simulink model "Lab3SquareDrive"  (R2024a)
settings: Solver=FixedStepDiscrete  StartTime=0.0  StopTime=90  FixedStep=0.01  RelTol=1e-3
undefined symbols (not defined in the file): DiscIntNeverNeededParam
libraries: mobileRoboticsTrainingLib x1
settings Model: PacingRate=5  Creator=Beast  LastModifiedBy=Beast

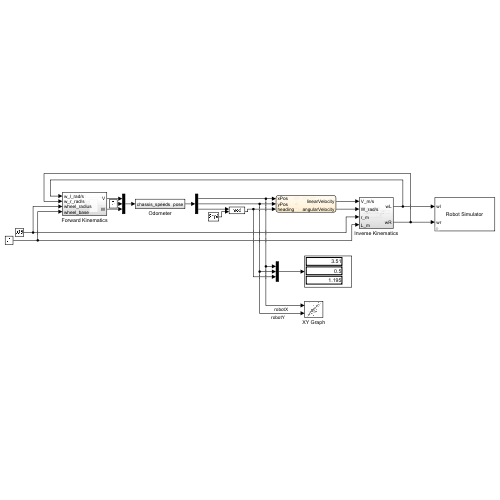
[thumbnail: Simulink's stored preview of the top-level diagram]
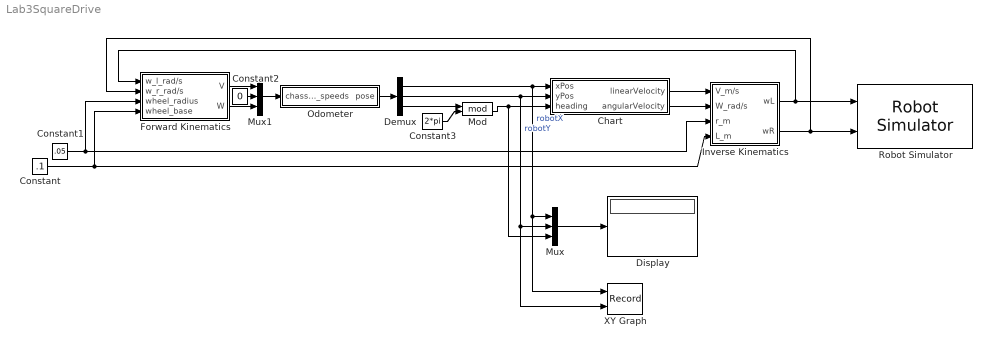
== system Lab3SquareDrive ==
  Chart : Stateflow chart  TreatAsAtomicUnit=on
  Constant : Constant  Value=.1
  Constant1 : Constant  Value=.05
  Constant2 : Constant  Value=0
  Constant3 : Constant  Value=2*pi
  Demux : Demux  Outputs=3
  Display : Display
  Forward Kinematics : Subsystem
  Inverse Kinematics : Subsystem
  Mod : Math  Operator=mod
  Mux : Mux  Inputs=3
  Mux1 : Mux  Inputs=3
  Odometer : Subsystem
  Robot Simulator : mobileRoboticsTrainingLib/Robot Simulator  Priority=99  mapVar=[]  startX=.5  startY=.5  startTheta=0  axleLength=0.1  wheelR=0.05
  XY Graph : Record  FileSettingsInternal="{\"entries\":[{\"content\":{\"excelSettings\":{\"content\":{},\"type\":\"Streamout.ExcelSettings\"}},\"type\":\"Streamout.FileSettingStorage\",\"uuid\":\"\"}],\"packageUris\":[\"http:\\/\\/schema.mathworks.com\\/mf0\\/streamout_blocks\\/R2020a\"],\"version\":\"1.0\"}"  Layout=[1 1]  SignalsInternal="{\"entries\":[{\"content\":{\"signals\":[{\"content\":{\"blockPath\":[],\"dimensions\":[1],\"domain\":\"\",\"lineColor\":\"#a2142f\",\"plots\":[ 1 ],\"port\":1,\"sid\":[\"\"],\"signalID\":1,\"signalName\":\"robotX\"},\"type\":\"RecordBlkView.Signal\",\"uuid\":\"\"},{\"content\":{\"blockPath\":[],\"dimensions\":[1],\"domain\":\"\",\"lineColor\":\"#139fff\",\"plots\":[ 1 ],\"port\":2,\"sid\":[\"\"],\"signalID\":2,\"signalName\":\"robotY\"},\"type\":\"RecordBlkView.Signal\",\"uuid\":\"\"}]},\"type\":\"RecordBlkView.InputSignals\",\"uuid\":\"\"}],\"packageUris\":[\"http:\\/\\/schema.mathworks.com\\/mf0\\/streamout_blocks\\/R2020a\"],\"version\":\"1.0\"}"  VisualizationBindings="{\"xyplotplugin\":{\"info\":[{\"series\":[{\"bindingParametersList\":[{\"parameter\":\"X-Axis\",\"signalID\":1,\"signalName\":\"robotX\"},{\"parameter\":\"Y-Axis\",\"signalID\":2,\"signalName\":\"robotY\"}],\"seriesID\":0}],\"subplotID\":1}]}}"  CompatibilityTag=XY
  wires:
  Chart/1(linearVelocity) -> Inverse Kinematics/1(V_m/s)
  Chart/2(angularVelocity) -> Inverse Kinematics/2(W_rad/s)
  Constant/1 -> Forward Kinematics/4(wheel_base), Inverse Kinematics/4(L_m)
  Constant1/1 -> Forward Kinematics/3(wheel_radius), Inverse Kinematics/3(r_m)
  Demux/1 -> XY Graph/1, Mux/1, Chart/1(xPos)  "robotX"
  Forward Kinematics/1(V) -> Mux1/1
  Forward Kinematics/2(W) -> Mux1/3
  Demux/2 -> XY Graph/2, Mux/2, Chart/2(yPos)  "robotY"
  Mux/1 -> Display/1
  Mux1/1 -> Odometer/1(chassis_speeds)
  Odometer/1(pose) -> Demux/1
  Constant2/1 -> Mux1/2
  Inverse Kinematics/1(wL) -> Forward Kinematics/1(w_l_rad/s), Robot Simulator/1
  Inverse Kinematics/2(wR) -> Forward Kinematics/2(w_r_rad/s), Robot Simulator/2
  Constant3/1 -> Mod/2
  Mod/1 -> Mux/3, Chart/3(heading)
  Demux/3 -> Mod/1

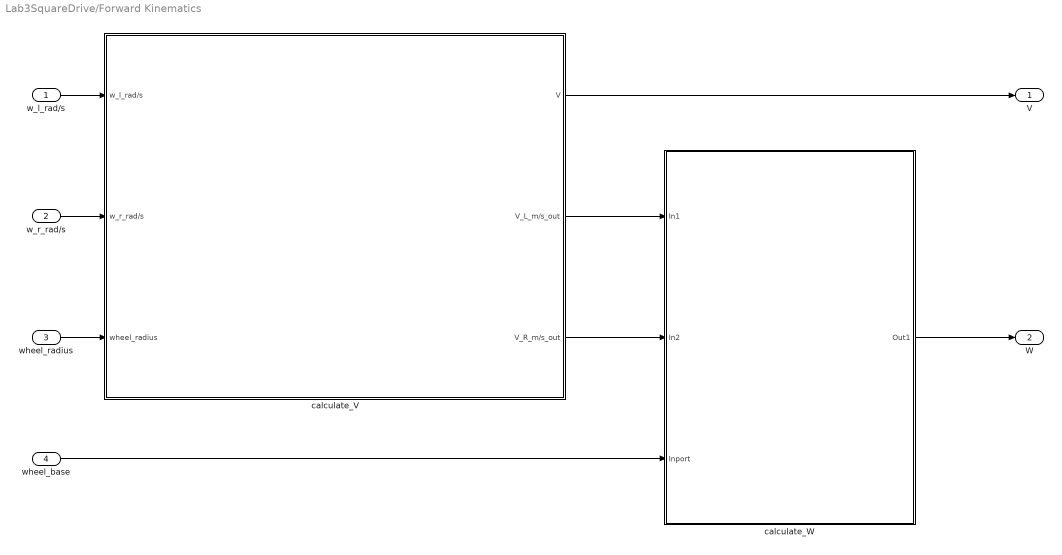
== system Lab3SquareDrive/Forward Kinematics ==
  w_l_rad/s : Inport
  w_r_rad/s : Inport  Port=2
  wheel_radius : Inport  Port=3
  wheel_base : Inport  Port=4
  calculate_V : Subsystem
  calculate_W : Subsystem
  V : Outport
  W : Outport  Port=2
  wires:
  calculate_V/1(V) -> V/1
  w_r_rad/s/1 -> calculate_V/2(w_r_rad/s)
  w_l_rad/s/1 -> calculate_V/1(w_l_rad/s)
  calculate_V/2(V_L_m/s_out) -> calculate_W/1(In1)
  calculate_W/1(Out1) -> W/1
  calculate_V/3(V_R_m/s_out) -> calculate_W/2(In2)
  wheel_radius/1 -> calculate_V/3(wheel_radius)
  wheel_base/1 -> calculate_W/3(Inport)

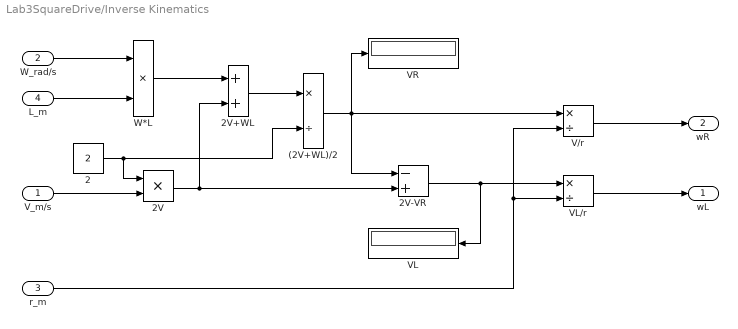
== system Lab3SquareDrive/Inverse Kinematics ==
  V_m/s : Inport
  W_rad/s : Inport  Port=2
  r_m : Inport  Port=3
  L_m : Inport  Port=4
  (2V+WL)/2 : Product  Inputs=*/
  2 : Constant  Value=2
  2V : Product
  2V+WL : Sum
  2V-VR : Sum  Inputs=-+
  V/r : Product  Inputs=*/
  VL : Display
  VL/r : Product  Inputs=*/
  VR : Display
  W*L : Product
  wL : Outport
  wR : Outport  Port=2
  wires:
  2/1 -> 2V/1, (2V+WL)/2/2
  W*L/1 -> 2V+WL/1
  (2V+WL)/2/1 -> 2V-VR/1, V/r/1, VR/1
  r_m/1 -> V/r/2, VL/r/2
  2V-VR/1 -> VL/r/1, VL/1
  2V/1 -> 2V+WL/2, 2V-VR/2
  VL/r/1 -> wL/1
  2V+WL/1 -> (2V+WL)/2/1
  V/r/1 -> wR/1
  V_m/s/1 -> 2V/2
  W_rad/s/1 -> W*L/1
  L_m/1 -> W*L/2

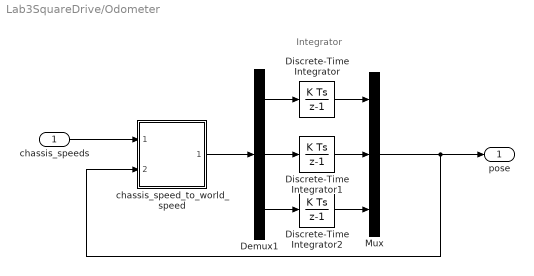
== system Lab3SquareDrive/Odometer ==
  note: Integrator
  chassis_speeds : Inport
  Demux1 : Demux  Outputs=3
  Discrete-Time Integrator : DiscreteIntegrator  InitialCondition=.5  SampleTime=-1  ICPrevOutput=DiscIntNeverNeededParam  ICPrevScaledInput=DiscIntNeverNeededParam
  Discrete-Time Integrator1 : DiscreteIntegrator  InitialCondition=.5  SampleTime=-1  ICPrevOutput=DiscIntNeverNeededParam  ICPrevScaledInput=DiscIntNeverNeededParam
  Discrete-Time Integrator2 : DiscreteIntegrator  SampleTime=-1  ICPrevOutput=DiscIntNeverNeededParam  ICPrevScaledInput=DiscIntNeverNeededParam
  Mux : Mux  Inputs=3
  chassis_speed_to_world_speed : Subsystem
  pose : Outport  VectorParamsAs1DForOutWhenUnconnected=off
  wires:
  Discrete-Time Integrator/1 -> Mux/1
  Demux1/2 -> Discrete-Time Integrator1/1
  Discrete-Time Integrator2/1 -> Mux/3
  Mux/1 -> chassis_speed_to_world_speed/2(last_pose), pose/1
  Demux1/3 -> Discrete-Time Integrator2/1
  Discrete-Time Integrator1/1 -> Mux/2
  Demux1/1 -> Discrete-Time Integrator/1
  chassis_speed_to_world_speed/1(global_velocity) -> Demux1/1
  chassis_speeds/1 -> chassis_speed_to_world_speed/1(robot_velocity)

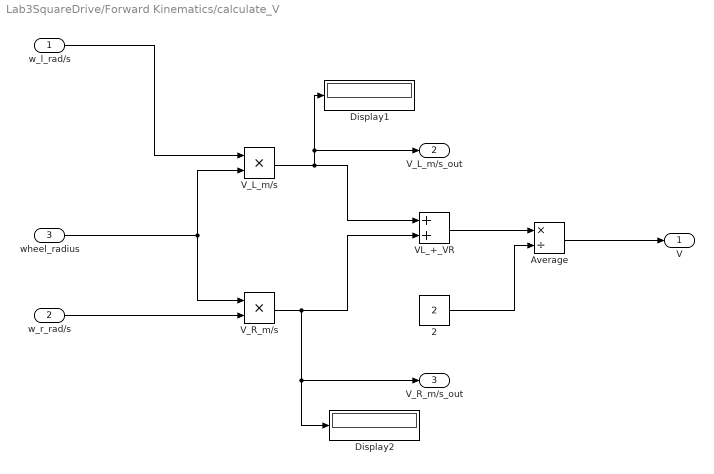
== system Lab3SquareDrive/Forward Kinematics/calculate_V ==
  w_l_rad/s : Inport
  w_r_rad/s : Inport  Port=2
  wheel_radius : Inport  Port=3
  2 : Constant  Value=2
  Average : Product  Inputs=*/
  Display1 : Display
  Display2 : Display
  VL_+_VR : Sum
  V_L_m/s : Product
  V_R_m/s : Product
  V : Outport
  V_L_m/s_out : Outport  Port=2
  V_R_m/s_out : Outport  Port=3
  wires:
  w_r_rad/s/1 -> V_R_m/s/2
  VL_+_VR/1 -> Average/1
  wheel_radius/1 -> V_L_m/s/2, V_R_m/s/1
  V_L_m/s/1 -> Display1/1, V_L_m/s_out/1, VL_+_VR/1
  V_R_m/s/1 -> V_R_m/s_out/1, Display2/1, VL_+_VR/2
  2/1 -> Average/2
  w_l_rad/s/1 -> V_L_m/s/1
  Average/1 -> V/1

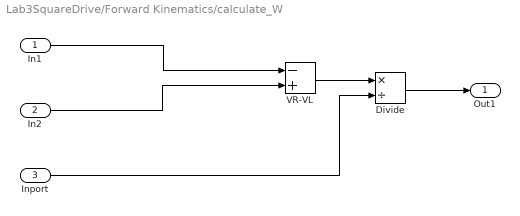
== system Lab3SquareDrive/Forward Kinematics/calculate_W ==
  In1 : Inport
  In2 : Inport  Port=2
  Inport : Inport  Port=3
  Divide : Product  Inputs=*/
  VR-VL : Sum  Inputs=-+
  Out1 : Outport
  wires:
  Inport/1 -> Divide/2
  VR-VL/1 -> Divide/1
  In2/1 -> VR-VL/2
  In1/1 -> VR-VL/1
  Divide/1 -> Out1/1

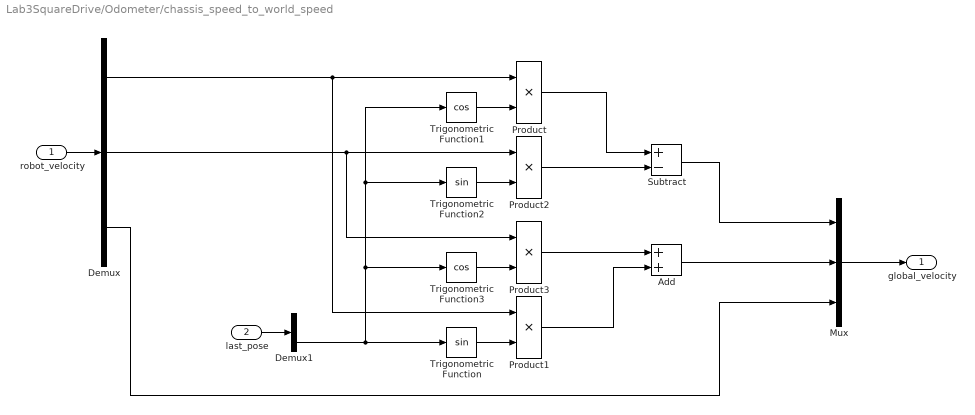
== system Lab3SquareDrive/Odometer/chassis_speed_to_world_speed ==
  robot_velocity : Inport
  last_pose : Inport  Port=2
  Add : Sum
  Demux : Demux  Outputs=3
  Demux1 : Demux  Outputs=3
  Mux : Mux  Inputs=3
  Product{,1..3} (4 alike) : Product
  Subtract : Sum  Inputs=+-
  Trigonometric Function : Trigonometry
  Trigonometric Function1 : Trigonometry  Operator=cos
  Trigonometric Function2 : Trigonometry
  Trigonometric Function3 : Trigonometry  Operator=cos
  global_velocity : Outport  VectorParamsAs1DForOutWhenUnconnected=off
  wires:
  Demux1/3 -> Trigonometric Function1/1, Trigonometric Function2/1, Trigonometric Function3/1, Trigonometric Function/1
  Trigonometric Function3/1 -> Product3/2
  Trigonometric Function/1 -> Product1/2
  robot_velocity/1 -> Demux/1
  Product1/1 -> Add/2
  Product2/1 -> Subtract/2
  Product/1 -> Subtract/1
  Demux/3 -> Mux/3
  Add/1 -> Mux/2
  Trigonometric Function1/1 -> Product/2
  Subtract/1 -> Mux/1
  Demux/1 -> Product/1, Product1/1
  Product3/1 -> Add/1
  Demux/2 -> Product3/1, Product2/1
  Mux/1 -> global_velocity/1
  Trigonometric Function2/1 -> Product2/2
  last_pose/1 -> Demux1/1

== stateflow chart Lab3SquareDrive/Chart ==
  state TurnLeft2
    entry:
    targetHeading = 1.5 * pi;
    linearVelocity = 0;
    angularVelocity = .5;
  state DriveLeft
    entry:
    targetX = xPos - 3;
    linearVelocity = 1;
    angularVelocity = 0;
  state TurnLeft1
    entry:
    targetHeading = pi;
    linearVelocity = 0;
    angularVelocity = .5;
  state DriveDown
    entry:
    targetY = yPos - 3;
    linearVelocity = 1;
    angularVelocity = 0;
  state DriveUp
    entry:
    targetY = yPos + 3;
    linearVelocity = 1;
    angularVelocity = 0;
  state TurnLeft3
    entry:
    targetHeading = 0;
    linearVelocity = 0;
    angularVelocity = .5;
  state DriveRight
    entry:
    targetX = xPos + 3;
    linearVelocity = 1;
    angularVelocity = 0;
  state TurnLeft
    entry:
    targetHeading = .5 * pi;
    linearVelocity = 0;
    angularVelocity = .5;
  DriveLeft -> TurnLeft2 : [xPos <= targetX]
  TurnLeft1 -> DriveLeft : [abs(heading - targetHeading) <= .01]
  TurnLeft2 -> DriveDown : [abs(heading - targetHeading) <= .01]
  DriveUp -> TurnLeft1 : [yPos >= targetY]
  DriveDown -> TurnLeft3 : [yPos <= targetY]
  TurnLeft -> DriveUp : [abs(heading - targetHeading) <= .01]
  (default) -> DriveRight
  TurnLeft3 -> DriveRight : [abs(heading - targetHeading) <= .01]
  DriveRight -> TurnLeft : [xPos >= targetX]
  data: xPos input; yPos input; linearVelocity output; heading input; targetHeading local; angularVelocity output; targetX local; targetY local
